simulink model "multilevelsimple"  (Simulink 7.4)
settings: Solver=ode45  StartTime=0.0  StopTime=0.1  RelTol=1e-3
libraries: powerlib x19
settings Model: Creator=balraj  LastModifiedBy=VIJAY
settings DebuggingCC: StrictBusMsg=ErrorLevel1

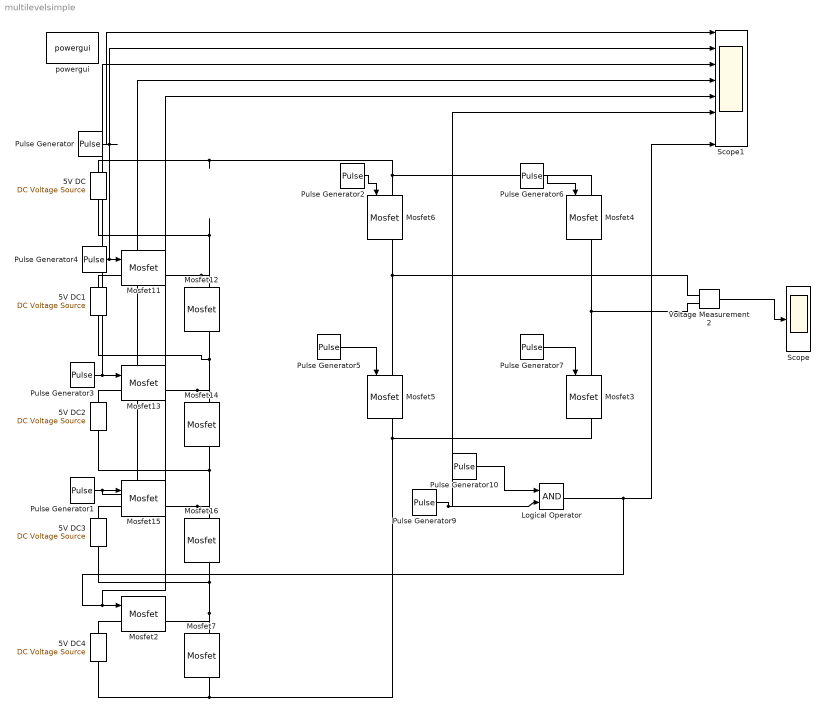
== system multilevelsimple ==
  5V DC{,1..4} (5 alike) : powerlib/Electrical Sources/DC Voltage Source  DialogController=POWERSYS.PowerSysDialog  SystemSampleTime=-1  Amplitude=50  Measurements=None
  Logical Operator : Logic  AllPortsSameDT=off  OutDataTypeMode=boolean  LogicDataType=fixdt(0, 8)  OutDataTypeStr=boolean
  Mosfet{2..7,11..16} (12 alike) : powerlib/Power Electronics/Mosfet  DialogController=POWERSYS.PowerSysDialog  SystemSampleTime=-1  Ron=0.1  Lon=0  Rd=0.01  Vfd=0  IC=0  Rs=1e5  Cs=inf  Measurements=on
  Pulse Generator : DiscretePulseGenerator  PulseType=Time based  Amplitude=5  Period=.01  PulseWidth=90  PhaseDelay=.0005  SampleTime=1
  Pulse Generator1 : DiscretePulseGenerator  PulseType=Time based  Amplitude=5  Period=.01  PulseWidth=30  PhaseDelay=.0035  SampleTime=1
  Pulse Generator10 : DiscretePulseGenerator  PulseType=Time based  Amplitude=5  Period=.01  PulseWidth=10  PhaseDelay=.0045  SampleTime=1
  Pulse Generator2 : DiscretePulseGenerator  PulseType=Time based  Amplitude=5  Period=.02  PulseWidth=45  PhaseDelay=0.0005  SampleTime=1
  Pulse Generator3 : DiscretePulseGenerator  PulseType=Time based  Amplitude=5  Period=.01  PulseWidth=50  PhaseDelay=.0025  SampleTime=1
  Pulse Generator4 : DiscretePulseGenerator  PulseType=Time based  Amplitude=5  Period=.01  PulseWidth=70  PhaseDelay=.0015  SampleTime=1
  Pulse Generator5 : DiscretePulseGenerator  PulseType=Time based  Amplitude=5  Period=.02  PulseWidth=45  PhaseDelay=.0105  SampleTime=1
  Pulse Generator6 : DiscretePulseGenerator  PulseType=Time based  Amplitude=5  Period=.02  PulseWidth=45  PhaseDelay=.0105  SampleTime=1
  Pulse Generator7 : DiscretePulseGenerator  PulseType=Time based  Amplitude=5  Period=.02  PulseWidth=45  PhaseDelay=.0005  SampleTime=1
  Pulse Generator9 : DiscretePulseGenerator  PulseType=Time based  Amplitude=5  Period=.0005  PulseWidth=50  PhaseDelay=.00062  SampleTime=1
  Scope : Scope
      settings: YMin=-260  YMax=260
  Scope1 : Scope  NumInputPorts=8
      settings: YMin=-0~0~-0~-0~-0~-0~-0~-0  YMax=6~6~6~6~6~6~6~5
  Voltage Measurement2 : powerlib/Measurements/Voltage Measurement  DialogController=POWERSYS.PowerSysDialog  SystemSampleTime=-1  PhasorSimulation=off  OutputType=Complex  PSBequivalent=0
  powergui : powerlib/powergui  Priority=1  SystemSampleTime=-1  SimulationMode=Continuous  SampleTime=50e-6  frequency=60  SPID=off  DisableSnubberDevices=off  DisableRonSwitches=off  DisableVfSwitches=off  SwTol=0  Interpol=off  frequencyindice=0  echomessages=off  HookPort=off  DisplayEquations=off  FunctionMessages=off  EnableUseOfTLC=off  x0status=blocks  RestoreLinks=warning  Frange=[0:2:500]  Ylog=off  Xlog=on  ShowGrid=off  save=off  variable=ZData  ZoomFFT=off  StartTime=0.0  cycles=1  DisplayStyle=1  fundamental=60  FreqAxis=off  MaxFrequency=1000  frequencyindicesteady=1  RmsSteady=1  display=off  Ts=0  methode=off
  wires:
  Pulse Generator/1 -> Scope1/1
  Pulse Generator4/1 -> Mosfet11/1, Scope1/2
  Pulse Generator2/1 -> Mosfet6/1
  Pulse Generator5/1 -> Mosfet5/1
  Pulse Generator7/1 -> Mosfet3/1
  Pulse Generator6/1 -> Mosfet4/1
  Voltage Measurement2/1 -> Scope/1
  Pulse Generator3/1 -> Mosfet13/1, Scope1/3
  Pulse Generator1/1 -> Scope1/4, Mosfet15/1
  Pulse Generator10/1 -> Logical Operator/1
  Pulse Generator9/1 -> Scope1/6, Logical Operator/2
  Logical Operator/1 -> Scope1/8, Mosfet2/1, Scope1/5
  connections:
  5V DC/RConn1 -- Mosfet6/LConn1 -- Mosfet4/LConn1
  5V DC1/RConn1 -- Mosfet11/LConn1
  Mosfet11/RConn1 -- Mosfet12/LConn1 -- 5V DC/LConn1
  5V DC2/RConn1 -- Mosfet13/LConn1
  Mosfet12/RConn1 -- Mosfet13/RConn1 -- Mosfet14/LConn1 -- 5V DC1/LConn1
  5V DC3/RConn1 -- Mosfet15/LConn1
  Mosfet16/LConn1 -- Mosfet14/RConn1 -- 5V DC2/LConn1 -- Mosfet15/RConn1
  Mosfet6/RConn1 -- Mosfet5/LConn1 -- Voltage Measurement2/LConn1
  Mosfet3/LConn1 -- Mosfet4/RConn1 -- Voltage Measurement2/LConn2
  Mosfet7/LConn1 -- 5V DC3/LConn1 -- Mosfet16/RConn1 -- Mosfet2/RConn1
  5V DC4/RConn1 -- Mosfet2/LConn1
  Mosfet7/RConn1 -- Mosfet5/RConn1 -- Mosfet3/RConn1 -- 5V DC4/LConn1
